simulink subsystem "USIF_LED_ColorCode"  (R2022b)
settings: Solver=VariableStepAuto  StartTime=0.0  StopTime=10.0  RelTol=1e-3
libraries: simulink x4, mbd_mpc574x_ec_toolbox x3
settings Model: Creator=MAAM  LastModifiedBy=MAAM

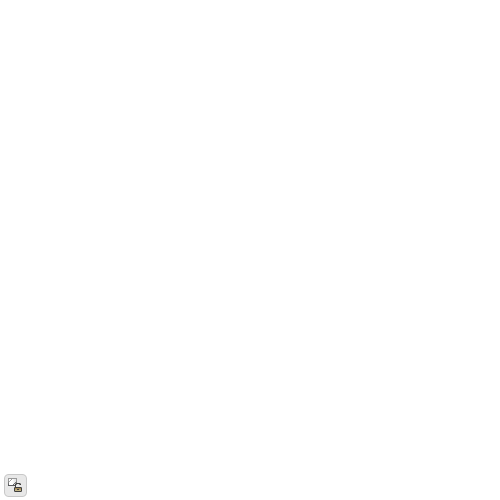
[thumbnail: Simulink's stored preview of the top-level diagram]
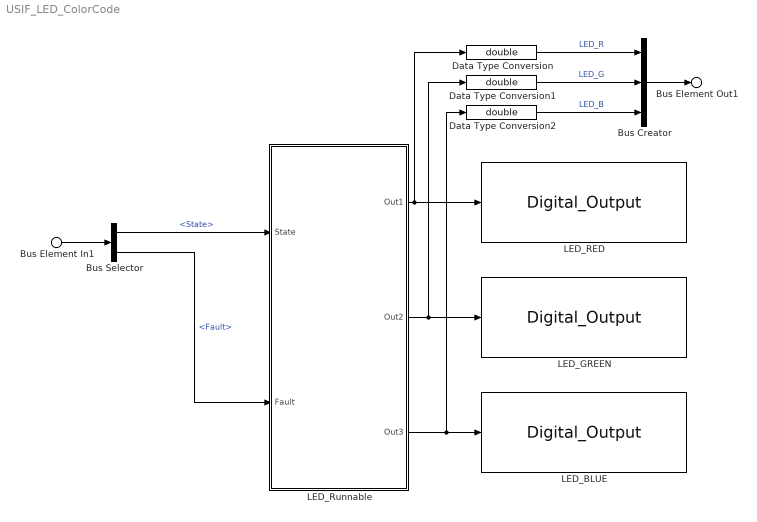
== system USIF_LED_ColorCode ==
  Bus Element In1 : Inport  PortName=SM_Status
  Bus Creator : BusCreator  Inputs=3
  Bus Selector : BusSelector  OutputSignals=State,Fault
  Data Type Conversion : DataTypeConversion  OutDataTypeStr=double  SaturateOnIntegerOverflow=off  RndMeth=Floor
  Data Type Conversion1 : DataTypeConversion  OutDataTypeStr=double  SaturateOnIntegerOverflow=off  RndMeth=Floor
  Data Type Conversion2 : DataTypeConversion  OutDataTypeStr=double  SaturateOnIntegerOverflow=off  RndMeth=Floor
  LED_BLUE : mbd_mpc574x_ec_toolbox/GPIO Blocks/Digital_Output  gpio_pin=PTC13: [SIUL2_GPIO45 | General Purpose IO PC[13]]  gpio_drive_strength=Disabled
  LED_GREEN : mbd_mpc574x_ec_toolbox/GPIO Blocks/Digital_Output  gpio_pin=PTC12: [SIUL2_GPIO44 | General Purpose IO PC[12]]  gpio_drive_strength=Disabled
  LED_RED : mbd_mpc574x_ec_toolbox/GPIO Blocks/Digital_Output  gpio_pin=PTC11: [SIUL2_GPIO43 | General Purpose IO PC[11]]  gpio_drive_strength=Disabled
  LED_Runnable : Subsystem
  Bus Element Out1 : Outport  PortName=LEDs
  wires:
  Data Type Conversion2/1 -> Bus Creator/3  "LED_B"
  Data Type Conversion1/1 -> Bus Creator/2  "LED_G"
  Data Type Conversion/1 -> Bus Creator/1  "LED_R"
  Bus Creator/1 -> Bus Element Out1/1
  LED_Runnable/3(Out3) -> Data Type Conversion2/1, LED_BLUE/1
  LED_Runnable/2(Out2) -> Data Type Conversion1/1, LED_GREEN/1
  LED_Runnable/1(Out1) -> Data Type Conversion/1, LED_RED/1
  Bus Element In1/1 -> Bus Selector/1
  Bus Selector/2 -> LED_Runnable/2(Fault)  "<Fault>"
  Bus Selector/1 -> LED_Runnable/1(State)  "<State>"

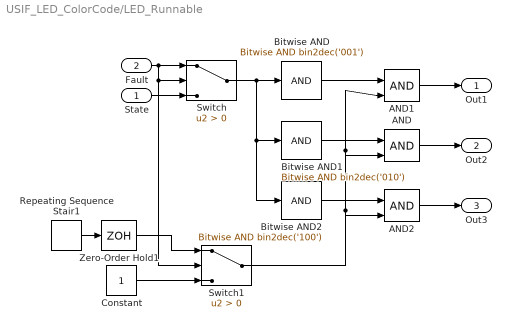
== system USIF_LED_ColorCode/LED_Runnable ==
  State : Inport
  Fault : Inport  Port=2
  AND : Logic  IconShape=distinctive  AllPortsSameDT=off  OutDataTypeStr=boolean
  AND1 : Logic  IconShape=distinctive  AllPortsSameDT=off  OutDataTypeStr=boolean
  AND2 : Logic  IconShape=distinctive  AllPortsSameDT=off  OutDataTypeStr=boolean
  Bitwise AND : simulink/Logic and Bit Operations/Bitwise Operator  logicop=AND  UseBitMask=on  BitMask=bin2dec('001')  BitMaskRealWorld=Stored Integer
      settings: LibrarySourceBlock=|
      | simulink/Quick Insert/Logic and Bit
      | Operations/Bitwise AND
  Bitwise AND1 : simulink/Logic and Bit Operations/Bitwise Operator  logicop=AND  UseBitMask=on  BitMask=bin2dec('010')  BitMaskRealWorld=Stored Integer
      settings: LibrarySourceBlock=|
      | simulink/Quick Insert/Logic and Bit
      | Operations/Bitwise AND
  Bitwise AND2 : simulink/Logic and Bit Operations/Bitwise Operator  logicop=AND  UseBitMask=on  BitMask=bin2dec('100')  BitMaskRealWorld=Stored Integer
      settings: LibrarySourceBlock=|
      | simulink/Quick Insert/Logic and Bit
      | Operations/Bitwise AND
  Constant : Constant  OutDataTypeStr=uint8
  Repeating Sequence Stair1 : simulink/Sources/Repeating Sequence Stair  OutValues=[0 1].'  tsamp=-1  OutMin=[]  OutMax=[]  OutDataTypeStr=uint8  OutputDataTypeScalingMode=uint8  OutDataType=fixdt(0,8)  ConRadixGroup=Best Precision: Vector-wise  OutScaling=2^-12
  Switch : Switch  Criteria=u2 > Threshold  SaturateOnIntegerOverflow=off  InputSameDT=off
  Switch1 : Switch  Criteria=u2 > Threshold  SaturateOnIntegerOverflow=off  InputSameDT=off
  Zero-Order Hold1 : ZeroOrderHold  SampleTime=0.1
  Out1 : Outport
  Out2 : Outport  Port=2
  Out3 : Outport  Port=3
  wires:
  Bitwise AND1/1 -> AND/1
  Switch1/1 -> AND2/2, AND1/2, AND/2
  Switch/1 -> Bitwise AND/1, Bitwise AND1/1, Bitwise AND2/1
  Fault/1 -> Switch/1, Switch/2, Switch1/2
  Repeating Sequence Stair1/1 -> Zero-Order Hold1/1
  AND2/1 -> Out3/1
  AND1/1 -> Out1/1
  State/1 -> Switch/3
  Constant/1 -> Switch1/3
  AND/1 -> Out2/1
  Bitwise AND/1 -> AND1/1
  Bitwise AND2/1 -> AND2/1
  Zero-Order Hold1/1 -> Switch1/1
